simulink model "Sample_HardThreshold"  (R2020a)
settings: Solver=VariableStepAuto  StartTime=0  StopTime=1  RelTol=1e-3
model workspace (MAT data in the model file):
  a = 0
values from neighbouring files (symbols this model uses):
  fs = 30000    [run_Sample_HardThreshold.m]
  refractory = 10^-3    (= 0.001)    [run_Sample_HardThreshold.m]
  th = [-70]    [run_Sample_HardThreshold.m]
libraries: dspfdesign x2, simulink x2, dspswit3 x1, hdlsllib x1
settings Model: Creator=sbuccelli  LastModifiedBy=diflo
settings DebuggingCC: SignalRangeChecking=warning

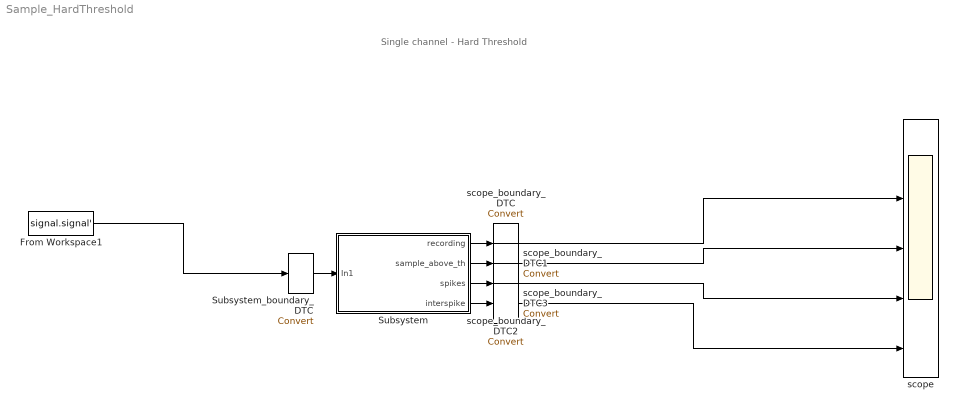
== system Sample_HardThreshold ==
  note: Single channel - Hard Threshold
  From Workspace1 : FromWorkspace  VariableName=signal.signal'  SampleTime=1/fs
  Subsystem : Subsystem
  Subsystem_boundary_DTC : DataTypeConversion  SaturateOnIntegerOverflow=on  RndMeth=Zero
  scope : Scope  NumInputPorts=5
  scope_boundary_DTC{,1..3} (4 alike) : DataTypeConversion  SaturateOnIntegerOverflow=on  RndMeth=Zero
  wires:
  From Workspace1/1 -> Subsystem_boundary_DTC/1
  Subsystem_boundary_DTC/1 -> Subsystem/1(In1)
  Subsystem/1(recording) -> scope_boundary_DTC/1
  scope_boundary_DTC/1 -> scope/2
  Subsystem/2(sample_above_th) -> scope_boundary_DTC1/1
  scope_boundary_DTC1/1 -> scope/3
  Subsystem/3(spikes) -> scope_boundary_DTC2/1
  scope_boundary_DTC2/1 -> scope/4
  Subsystem/4(interspike) -> scope_boundary_DTC3/1
  scope_boundary_DTC3/1 -> scope/5

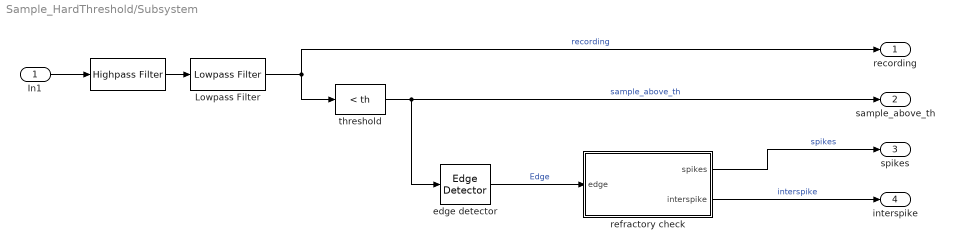
== system Sample_HardThreshold/Subsystem ==
  In1 : Inport
  " " : dspfdesign/Highpass Filter  FilterType=IIR  DesignForMinimumOrder=on  FilterOrder=50  StopbandFrequency=1  PassbandFrequency=300  StopbandAttenuation=80  PassbandRipple=0.1  InheritSampleRate=off  SampleRate=fs  SimulateUsing=Interpreted execution  roundingMode=Floor  coeffsDataTypeStr=fixdt(1,16)
  Lowpass Filter : dspfdesign/Lowpass Filter  FilterType=IIR  DesignForMinimumOrder=on  FilterOrder=3  PassbandFrequency=3500  StopbandFrequency=8500  PassbandRipple=0.1  StopbandAttenuation=80  InheritSampleRate=off  SampleRate=fs  SimulateUsing=Interpreted execution  roundingMode=Floor  coeffsDataTypeStr=fixdt(1,16)
  "edge detector " : dspswit3/Edge Detector  InputProcessing=Columns as channels (frame based)
      settings: SourceProductBaseCode=DS
  refractory check : Subsystem
  threshold : simulink/Logic and Bit Operations/Compare To Constant  relop=<  const=th  OutDataTypeStr=boolean
  recording : Outport
  sample_above_th : Outport  Port=2
  spikes : Outport  Port=3
  interspike : Outport  Port=4
  wires:
  threshold/1 -> sample_above_th/1, "edge detector "/1  "sample_above_th"
  "edge detector "/1 -> refractory check/1("edge  ")  "Edge"
  refractory check/2(interspike) -> interspike/1  "interspike"
  " "/1 -> Lowpass Filter/1
  Lowpass Filter/1 -> recording/1, threshold/1  "recording"
  In1/1 -> " "/1
  refractory check/1(spikes) -> spikes/1  "spikes"

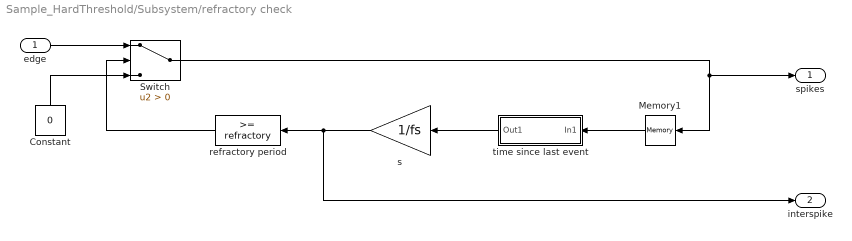
== system Sample_HardThreshold/Subsystem/refractory check ==
  "edge  " : Inport
  Constant : Constant  Value=0
  Memory1 : Memory  InheritSampleTime=on
  Switch : Switch  Criteria=u2 > Threshold
  refractory period : simulink/Logic and Bit Operations/Compare To Constant  relop=>=  const=refractory  OutDataTypeStr=boolean
  s : Gain  Gain=1/fs  ParamDataTypeStr=double
  time since last event : Subsystem
  spikes : Outport
  interspike : Outport  Port=2
  wires:
  "edge  "/1 -> Switch/1
  Memory1/1 -> time since last event/1(In1)
  time since last event/1(Out1) -> s/1
  Constant/1 -> Switch/3
  s/1 -> refractory period/1, interspike/1
  Switch/1 -> spikes/1, Memory1/1
  refractory period/1 -> Switch/2

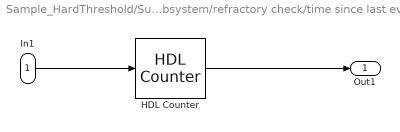
== system Sample_HardThreshold/Subsystem/refractory check/time since last event ==
  In1 : Inport
  HDL Counter : hdlsllib/Sources/HDL Counter  CountType=Free running  CountInit=1  CountStep=1  CountMax=25  CountFromType=Initial value  CountFrom=1  CountResetPort=on  CountLoadPort=off  CountEnbPort=off  CountDirPort=off  CountDataType=Unsigned  CountWordLen=32  CountFracLen=0  CountSampTime=1
  Out1 : Outport
  wires:
  In1/1 -> HDL Counter/1
  HDL Counter/1 -> Out1/1
